simulink model "Dynamic_Modelspeed"  (R2023a)
settings: Solver=ode4  StartTime=0.0  StopTime=1.5  FixedStep=Ts  RelTol=1e-3
InitFcn:
  | eval  SRM_Parameters ;
undefined symbols (not defined in the file): B, Curr_F_4Q_MH, di, DiscIntNeverNeededParam, I_peak, J, KD, KI, KP, sigbuilder_block, T_4Q_MH, Ts, Vdc
libraries: simulink x3, dspsigops x1
(part 5 of 5)

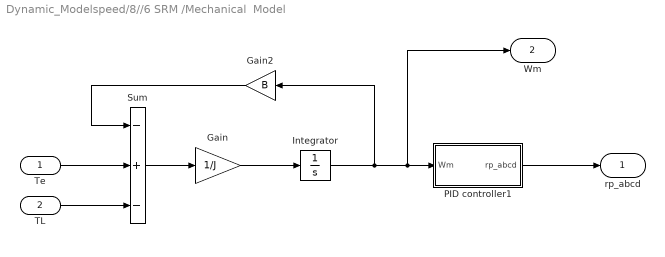
== system Dynamic_Modelspeed/8//6 SRM /Mechanical  Model ==
  Te : Inport
  TL : Inport  Port=2
  Gain : Gain  Gain=1/J
  Gain2 : Gain  Gain=B
  Integrator : Integrator
  PID controller1 : Subsystem
  Sum : Sum  Inputs=-+-
  rp_abcd : Outport
  Wm : Outport  Port=2
  wires:
  Sum/1 -> Gain/1
  Gain/1 -> Integrator/1
  TL/1 -> Sum/3
  Gain2/1 -> Sum/1
  PID controller1/1(rp_abcd) -> rp_abcd/1
  Te/1 -> Sum/2
  Integrator/1 -> Wm/1, PID controller1/1(Wm), Gain2/1

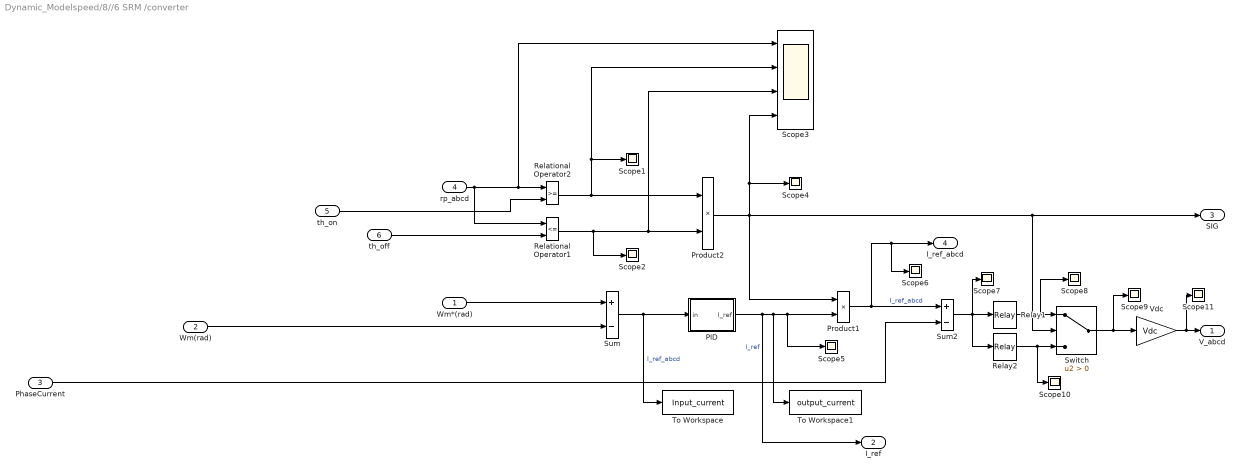
== system Dynamic_Modelspeed/8//6 SRM /converter ==
  Wm*(rad) : Inport
  Wm(rad) : Inport  Port=2
  PhaseCurrent : Inport  Port=3
  rp_abcd : Inport  Port=4
  th_on : Inport  Port=5
  th_off : Inport  Port=6
  PID : Subsystem
  Product1 : Product  OutDataTypeStr=double  SaturateOnIntegerOverflow=on
  Product2 : Product  OutDataTypeStr=double  SaturateOnIntegerOverflow=on
  Relational Operator1 : RelationalOperator  Operator=<=  OutDataTypeStr=fixdt(1,16)  InputSameDT=off
  Relational Operator2 : RelationalOperator  OutDataTypeStr=fixdt(1,16)  InputSameDT=off
  Relay1 : Relay  OnSwitchValue=di  OffSwitchValue=-di  OffOutputValue=-1  SampleTime=Ts
  Relay2 : Relay  OnSwitchValue=0.001  OffSwitchValue=-0.001  OffOutputValue=-1  SampleTime=Ts
  Scope{1..2,4..11} (10 alike) : Scope
  Scope3 : Scope  NumInputPorts=4
  Sum : Sum  Inputs=+-
  Sum2 : Sum  Inputs=+-  SaturateOnIntegerOverflow=on
  Switch : Switch  Criteria=u2 > Threshold  SaturateOnIntegerOverflow=off  InputSameDT=off
  To Workspace : ToWorkspace  VariableName=Input_current  SaveFormat=Timeseries  SampleTime=-1
      settings: Decimation=4
  To Workspace1 : ToWorkspace  VariableName=output_current  SaveFormat=Timeseries  SampleTime=-1
      settings: Decimation=4
  Vdc : Gain  Gain=Vdc
  V_abcd : Outport
  I_ref : Outport  Port=2
  SIG : Outport  Port=3
  I_ref_abcd : Outport  Port=4
  wires:
  Relational Operator1/1 -> Scope3/3, Product2/2, Scope2/1
  Relational Operator2/1 -> Scope3/2, Scope1/1, Product2/1
  rp_abcd/1 -> Relational Operator1/1, Scope3/1, Relational Operator2/1
  Product1/1 -> Scope6/1, I_ref_abcd/1, Sum2/1  "I_ref_abcd"
  PhaseCurrent/1 -> Sum2/2
  Product2/1 -> Product1/1, Scope3/4, Scope4/1, Switch/2, SIG/1
  Sum2/1 -> Scope7/1, Relay2/1, Relay1/1
  Vdc/1 -> Scope11/1, V_abcd/1
  Relay2/1 -> Scope10/1, Switch/3
  Switch/1 -> Scope9/1, Vdc/1
  Relay1/1 -> Scope8/1, Switch/1
  PID/1(I_ref) -> To Workspace1/1, Scope5/1, Product1/2, I_ref/1  "I_ref"
  Wm*(rad)/1 -> Sum/1
  Wm(rad)/1 -> Sum/2
  Sum/1 -> PID/1(in), To Workspace/1  "I_ref_abcd"
  th_off/1 -> Relational Operator1/2
  th_on/1 -> Relational Operator2/2

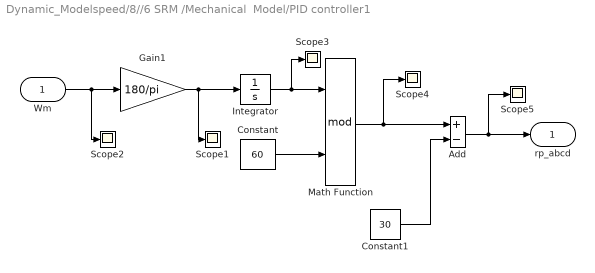
== system Dynamic_Modelspeed/8//6 SRM /Mechanical  Model/PID controller1 ==
  Wm : Inport
  Add : Sum  Inputs=+-
  Constant : Constant  Value=60
  Constant1 : Constant  Value=30
  Gain1 : Gain  Gain=180/pi  SaturateOnIntegerOverflow=on  OutDataTypeStr=Inherit: Same as input  ParamDataTypeStr=Inherit: Same as input
  Integrator : Integrator  InitialCondition=[0 -15 -30 -45]
  Math Function : Math  Operator=mod  SignedPower=on
  Scope{1..5} (5 alike) : Scope
  rp_abcd : Outport
  wires:
  Gain1/1 -> Scope1/1, Integrator/1
  Integrator/1 -> Scope3/1, Math Function/1
  Constant/1 -> Math Function/2
  Math Function/1 -> Scope4/1, Add/1
  Wm/1 -> Scope2/1, Gain1/1
  Add/1 -> Scope5/1, rp_abcd/1
  Constant1/1 -> Add/2

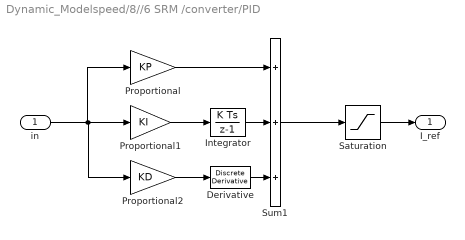
== system Dynamic_Modelspeed/8//6 SRM /converter/PID ==
  in : Inport
  " Derivative" : simulink/Discrete/Discrete Derivative  gainval=1.0  ICPrevScaledInput=0.0  OutMin=[]  OutMax=[]  OutDataType=fixdt(1, 16)  OutScaling=2^-10  DoSatur=off
  Integrator : DiscreteIntegrator  SampleTime=-1  ICPrevOutput=DiscIntNeverNeededParam  ICPrevScaledInput=DiscIntNeverNeededParam
  Proportional : Gain  Gain=KP  SaturateOnIntegerOverflow=on  OutDataTypeStr=Inherit: Same as input  ParamDataTypeStr=Inherit: Same as input
  Proportional1 : Gain  Gain=KI  SaturateOnIntegerOverflow=on  OutDataTypeStr=Inherit: Same as input  ParamDataTypeStr=Inherit: Same as input
  Proportional2 : Gain  Gain=KD  SaturateOnIntegerOverflow=on  OutDataTypeStr=Inherit: Same as input  ParamDataTypeStr=Inherit: Same as input
  Saturation : Saturate  UpperLimit=I_peak  LowerLimit=-I_peak
  Sum1 : Sum  Inputs=+++  InputSameDT=on  SaturateOnIntegerOverflow=on  OutDataTypeStr=Inherit: Same as first input
  I_ref : Outport
  wires:
  Integrator/1 -> Sum1/2
  Proportional/1 -> Sum1/1
  Sum1/1 -> Saturation/1
  Saturation/1 -> I_ref/1
  in/1 -> Proportional2/1, Proportional1/1, Proportional/1
  Proportional2/1 -> " Derivative"/1
  " Derivative"/1 -> Sum1/3
  Proportional1/1 -> Integrator/1
